simulink model "overview"  (R2016b)
settings: Solver=FixedStepAuto  StartTime=0.0  StopTime=1  FixedStep=0.00001  RelTol=1e-3
settings Model: Creator=Niirn  LastModifiedBy=Niirn

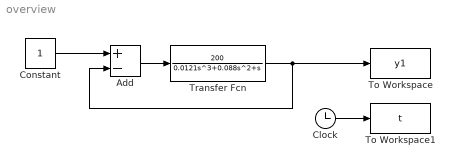
== system overview ==
  Add : Sum  Inputs=+-
  Clock : Clock
  Constant : Constant
  To Workspace : ToWorkspace  VariableName=y1  SampleTime=-1
  To Workspace1 : ToWorkspace  VariableName=t  SampleTime=-1
  Transfer Fcn : TransferFcn  Numerator=[200]  Denominator=[0.0121 0.088 1 0]
  wires:
  Transfer Fcn/1 -> To Workspace/1, Add/2
  Constant/1 -> Add/1
  Add/1 -> Transfer Fcn/1
  Clock/1 -> To Workspace1/1
